simulink model "cdnlink_lb_wide_15a"  (Simulink 8.5)
settings: Solver=ode45  StartTime=0.0  StopTime=10.0  RelTol=1e-3
undefined symbols (not defined in the file): des, gcbh
(part 2 of 3)

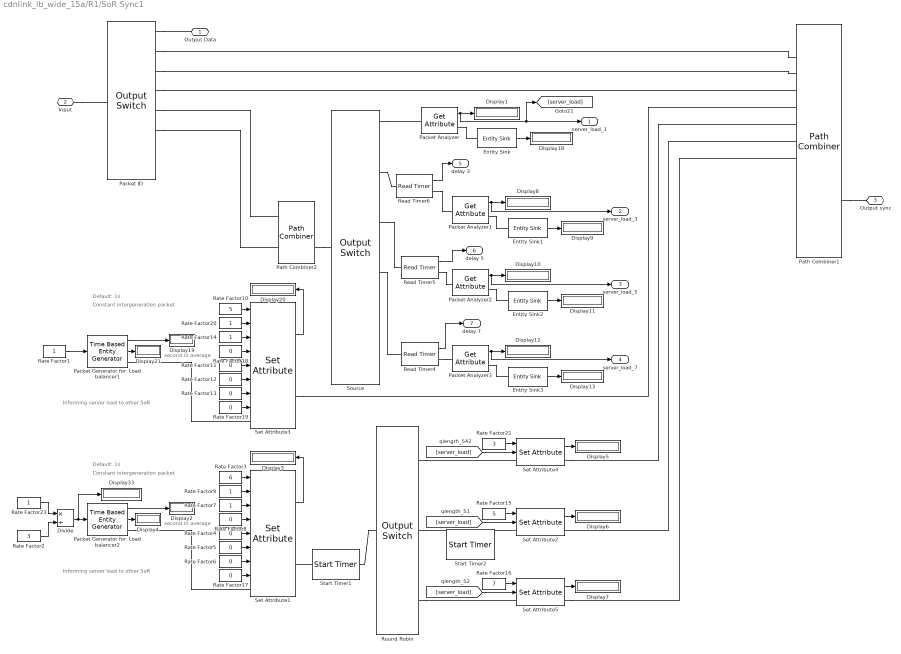
== system cdnlink_lb_wide_15a/R1/SoR Sync1 ==
  note: second in average
  note: Constant intergeneration packet
  note: Default: 1s
  note: Informing server load to other SoR
  note: second in average
  note: Constant intergeneration packet
  note: Default: 1s
  note: Informing server load to other SoR
  Display{1..13,18..21,33} (18 alike) : Display
  Divide : Product  Inputs=*/
  Entity Sink{,1..3} (4 alike) : EntitySink  StatNumberArrived=on
  Packet Analyzer : GetAttribute  AttributeName=av_load1  EvaluatedDefaultAttributeValue={ []}
      settings: OutputPortMap=o1
  Packet Analyzer1 : GetAttribute  AttributeName=server_load  EvaluatedDefaultAttributeValue={ []}
      settings: OutputPortMap=o1
  Packet Analyzer2 : GetAttribute  AttributeName=server_load  EvaluatedDefaultAttributeValue={ []}
      settings: OutputPortMap=o1
  Packet Analyzer3 : GetAttribute  AttributeName=server_load  EvaluatedDefaultAttributeValue={ []}
      settings: OutputPortMap=o1
  Packet Generator for  Load balancer1 : TimeBasedEntityGenerator  GenerateEntitiesUpon=Intergeneration time from port t  InitialSeed=6765331  Mean=0.05  EntityType=Standard  StatNumberDeparted=on  StatAverageIntergenerationTime=on
      settings: OutputPortMap=o0,o2
  Packet Generator for  Load balancer2 : TimeBasedEntityGenerator  GenerateEntitiesUpon=Intergeneration time from port t  InitialSeed=6765331  Mean=0.05  EntityType=Standard  StatNumberDeparted=on  StatAverageIntergenerationTime=on
      settings: OutputPortMap=o0,o2
  Packet ID : OutputSwitch  NumberOutputPorts=8  SwitchingCriterion=From attribute  AttributeName=packet_id
  Path Combiner1 : PathCombiner  NumberInputPorts=13  StatNumberDeparted=on
  Path Combiner2 : PathCombiner  NumberInputPorts=2  StatNumberDeparted=on
  Rate Factor{1,7,9,14,20,23} (6 alike) : Constant
  Rate Factor10 : Constant  Value=5
  Rate Factor{4..6,8,11..13,17..19} (10 alike) : Constant  Value=0
  Rate Factor15 : Constant  Value=5
  Rate Factor16 : Constant  Value=7
  Rate Factor2 : Constant  Value=3
  Rate Factor21 : Constant  Value=3
  Rate Factor3 : Constant  Value=6
  Read Timer4 : ReadTimer  TimerTag=id6  StatTimeElapsed=on
      settings: OutputPortMap=o2
  Read Timer5 : ReadTimer  TimerTag=id6  StatTimeElapsed=on
      settings: OutputPortMap=o2
  Read Timer6 : ReadTimer  TimerTag=id6  StatTimeElapsed=on
      settings: OutputPortMap=o2
  Round Robin : OutputSwitch  SwitchingCriterion=Round robin  AttributeName=source
  Set Attribute1 : SetAttribute  AttributeName=packet_id|reply|source|server_load|content_time|dest|hop_count|router_id  AttributeFrom=Signal port|Signal port|Signal port|Signal port|Signal port|Signal port|Signal port|Signal port  AttributeValue=1|1|1|1|1|1|1|1  AttributeTreatAsVector=1|1|1|1|1|1|1|1  StatNumberDeparted=on  EvaluatedAttributeValue={ [];[];[];[];[];[];[];[]}
      settings: InputPortMap=u0,u1,u2,u3,u4,u5,u6,u7
  Set Attribute2 : SetAttribute  AttributeName=dest|server_load  AttributeFrom=Signal port|Signal port  AttributeValue=1|1  AttributeTreatAsVector=1|1  StatNumberDeparted=on  EvaluatedAttributeValue={ [];[]}
      settings: InputPortMap=u0,u1
  Set Attribute3 : SetAttribute  AttributeName=packet_id|reply|source|server_load|content_time|dest|hop_count|router_id  AttributeFrom=Signal port|Signal port|Signal port|Signal port|Signal port|Signal port|Signal port|Signal port  AttributeValue=1|1|1|1|1|1|1|1  AttributeTreatAsVector=1|1|1|1|1|1|1|1  StatNumberDeparted=on  EvaluatedAttributeValue={ [];[];[];[];[];[];[];[]}
      settings: InputPortMap=u0,u1,u2,u3,u4,u5,u6,u7
  Set Attribute4 : SetAttribute  AttributeName=dest|server_load  AttributeFrom=Signal port|Signal port  AttributeValue=1|1  AttributeTreatAsVector=1|1  StatNumberDeparted=on  EvaluatedAttributeValue={ [];[]}
      settings: InputPortMap=u0,u1
  Set Attribute5 : SetAttribute  AttributeName=dest|server_load  AttributeFrom=Signal port|Signal port  AttributeValue=1|1  AttributeTreatAsVector=1|1  StatNumberDeparted=on  EvaluatedAttributeValue={ [];[]}
      settings: InputPortMap=u0,u1
  Source : OutputSwitch  NumberOutputPorts=11  SwitchingCriterion=From attribute  AttributeName=source
  Start Timer1 : StartTimer  TimerTag=id6
  Start Timer2 : StartTimer  TimerTag=id6
  Output Data : PMIOPort  Port=1  Side=Right
  Input : PMIOPort  Port=2  Side=Left
  Output sync : PMIOPort  Port=3  Side=Right
  server_load_1 : Outport
  server_load_3 : Outport  Port=2
  server_load_5 : Outport  Port=3
  server_load_7 : Outport  Port=4
  delay 3 : Outport  Port=5
  delay 5 : Outport  Port=6
  delay 7 : Outport  Port=7
  wires:
  Packet Generator for  Load balancer1/1 -> Display19/1
  Rate Factor14/1 -> Set Attribute3/3
  Rate Factor10/1 -> Set Attribute3/1
  Rate Factor20/1 -> Set Attribute3/2
  Packet Generator for  Load balancer1/2 -> Display21/1
  Rate Factor18/1 -> Set Attribute3/4
  Set Attribute3/1 -> Display20/1
  Rate Factor11/1 -> Set Attribute3/5
  Rate Factor12/1 -> Set Attribute3/6
  Rate Factor13/1 -> Set Attribute3/7
  Rate Factor1/1 -> Packet Generator for  Load balancer1/1
  Packet Analyzer/1 -> [server_load], server_load_1/1, Display1/1
  Entity Sink/1 -> Display18/1
  Packet Generator for  Load balancer2/1 -> Display2/1
  Rate Factor7/1 -> Set Attribute1/3
  Rate Factor3/1 -> Set Attribute1/1
  Rate Factor9/1 -> Set Attribute1/2
  Packet Generator for  Load balancer2/2 -> Display4/1
  Rate Factor8/1 -> Set Attribute1/4
  Set Attribute1/1 -> Display3/1
  Rate Factor4/1 -> Set Attribute1/5
  Rate Factor5/1 -> Set Attribute1/6
  Rate Factor6/1 -> Set Attribute1/7
  Rate Factor21/1 -> Set Attribute4/1
  Set Attribute4/1 -> Display5/1
  [server_load] -> Set Attribute4/2
  Rate Factor15/1 -> Set Attribute2/1
  Set Attribute2/1 -> Display6/1
  [server_load] -> Set Attribute2/2
  Rate Factor16/1 -> Set Attribute5/1
  Set Attribute5/1 -> Display7/1
  [server_load] -> Set Attribute5/2
  Packet Analyzer1/1 -> server_load_3/1, Display8/1
  Entity Sink1/1 -> Display9/1
  Packet Analyzer2/1 -> server_load_5/1, Display10/1
  Entity Sink2/1 -> Display11/1
  Packet Analyzer3/1 -> server_load_7/1, Display12/1
  Entity Sink3/1 -> Display13/1
  Rate Factor23/1 -> Divide/1
  Rate Factor2/1 -> Divide/2
  Divide/1 -> Packet Generator for  Load balancer2/1, Display33/1
  Rate Factor17/1 -> Set Attribute1/8
  Rate Factor19/1 -> Set Attribute3/8
  Read Timer6/1 -> delay 3/1
  Read Timer5/1 -> delay 5/1
  Read Timer4/1 -> delay 7/1
  connections:
  Packet Generator for  Load balancer1/RConn1 -- Set Attribute3/LConn1
  Packet ID/RConn5 -- Path Combiner2/LConn1
  Packet ID/RConn2 -- Path Combiner1/LConn2
  Packet ID/RConn3 -- Path Combiner1/LConn3
  Packet ID/RConn4 -- Path Combiner1/LConn4
  Set Attribute3/RConn1 -- Path Combiner1/LConn5
  Packet ID/RConn1 -- Output Data/RConn1
  Path Combiner1/RConn1 -- Output sync/RConn1
  Packet Analyzer/RConn1 -- Entity Sink/LConn1
  Source/RConn1 -- Packet Analyzer/LConn1
  Start Timer1/LConn1 -- Set Attribute1/RConn1
  Packet Generator for  Load balancer2/RConn1 -- Set Attribute1/LConn1
  Round Robin/RConn1 -- Set Attribute4/LConn1
  Round Robin/RConn2 -- Set Attribute2/LConn1
  Round Robin/RConn3 -- Set Attribute5/LConn1
  Packet Analyzer1/RConn1 -- Entity Sink1/LConn1
  Packet Analyzer2/RConn1 -- Entity Sink2/LConn1
  Packet Analyzer3/RConn1 -- Entity Sink3/LConn1
  Source/RConn5 -- Read Timer5/LConn1
  Path Combiner2/RConn1 -- Source/LConn1
  Packet ID/RConn6 -- Path Combiner2/LConn2
  Set Attribute4/RConn1 -- Path Combiner1/LConn6
  Path Combiner1/LConn7 -- Set Attribute2/RConn1
  Set Attribute5/RConn1 -- Path Combiner1/LConn8
  Input/RConn1 -- Packet ID/LConn1
  Round Robin/LConn1 -- Start Timer1/RConn1
  Read Timer4/RConn1 -- Packet Analyzer3/LConn1
  Source/RConn7 -- Read Timer4/LConn1
  Read Timer5/RConn1 -- Packet Analyzer2/LConn1
  Source/RConn3 -- Read Timer6/LConn1
  Read Timer6/RConn1 -- Packet Analyzer1/LConn1

== system cdnlink_lb_wide_15a/R3/ 1 ==
  note: Exponential Distribution
      | Service Rate Generator
  note: CDNlink-NS
  note: 830 packet/ second = 10 Mbps
      | for Router --> 500 Mbps = 830*10*5 = 41500
      | for Server --> 100 Mbps = 830*10 = 8300
  "  " : Subsystem  mask(Exponential Random Number Generator){seed=85274}
      mask prompts: seed "Initial seed"
      mask help: Output exponentially distributed random numbers with the input rate. Output is repeatable for a given seed.
      mask Display: disp('Exponential\n Distribution');
  Display1 : Display
  Display4 : Display
  Service time : Outport
  wires:
  "  "/1(Out1) -> Display1/1, Service time/1
  [router3] -> Display4/1, "  "/1(Arrival Rate)

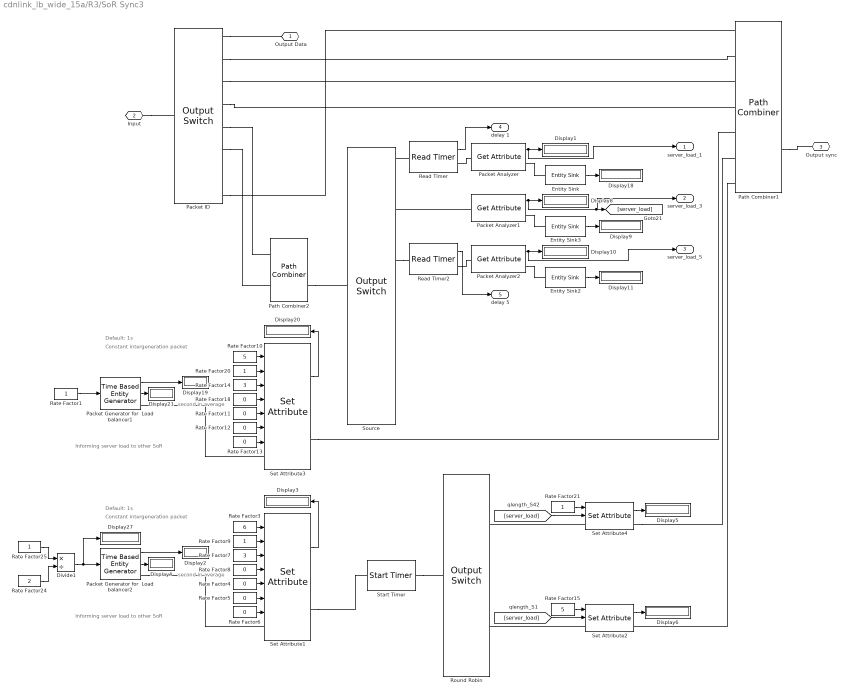
== system cdnlink_lb_wide_15a/R3/SoR Sync3 ==
  note: second in average
  note: Constant intergeneration packet
  note: Default: 1s
  note: Informing server load to other SoR
  note: second in average
  note: Constant intergeneration packet
  note: Default: 1s
  note: Informing server load to other SoR
  Display{1..6,8..11,18..21,27} (15 alike) : Display
  Divide1 : Product  Inputs=*/
  Entity Sink : EntitySink  StatNumberArrived=on
  Entity Sink2 : EntitySink  StatNumberArrived=on
  Entity Sink3 : EntitySink  StatNumberArrived=on
  Packet Analyzer : GetAttribute  AttributeName=server_load  EvaluatedDefaultAttributeValue={ []}
      settings: OutputPortMap=o1
  Packet Analyzer1 : GetAttribute  AttributeName=server_load  EvaluatedDefaultAttributeValue={ []}
      settings: OutputPortMap=o1
  Packet Analyzer2 : GetAttribute  AttributeName=server_load  EvaluatedDefaultAttributeValue={ []}
      settings: OutputPortMap=o1
  Packet Generator for  Load balancer1 : TimeBasedEntityGenerator  GenerateEntitiesUpon=Intergeneration time from port t  InitialSeed=6765331  Mean=0.05  EntityType=Standard  StatNumberDeparted=on  StatAverageIntergenerationTime=on
      settings: OutputPortMap=o0,o2
  Packet Generator for  Load balancer2 : TimeBasedEntityGenerator  GenerateEntitiesUpon=Intergeneration time from port t  InitialSeed=6765331  Mean=0.05  EntityType=Standard  StatNumberDeparted=on  StatAverageIntergenerationTime=on
      settings: OutputPortMap=o0,o2
  Packet ID : OutputSwitch  NumberOutputPorts=8  SwitchingCriterion=From attribute  AttributeName=packet_id
  Path Combiner1 : PathCombiner  NumberInputPorts=7  StatNumberDeparted=on
  Path Combiner2 : PathCombiner  NumberInputPorts=2  StatNumberDeparted=on
  Rate Factor{1,9,20..21,25} (5 alike) : Constant
  Rate Factor10 : Constant  Value=5
  Rate Factor{4..6,8,11..13,18} (8 alike) : Constant  Value=0
  Rate Factor14 : Constant  Value=3
  Rate Factor15 : Constant  Value=5
  Rate Factor24 : Constant  Value=2
  Rate Factor3 : Constant  Value=6
  Rate Factor7 : Constant  Value=3
  Read Timer : ReadTimer  TimerTag=id6  StatTimeElapsed=on
      settings: OutputPortMap=o2
  Read Timer2 : ReadTimer  TimerTag=id6  StatTimeElapsed=on
      settings: OutputPortMap=o2
  Round Robin : OutputSwitch  NumberOutputPorts=2  SwitchingCriterion=Round robin  AttributeName=source
  Set Attribute1 : SetAttribute  AttributeName=packet_id|reply|source|server_load|content_time|dest|hop_count  AttributeFrom=Signal port|Signal port|Signal port|Signal port|Signal port|Signal port|Signal port  AttributeValue=1|1|1|1|1|1|1  AttributeTreatAsVector=1|1|1|1|1|1|1  StatNumberDeparted=on  EvaluatedAttributeValue={ [];[];[];[];[];[];[]}
      settings: InputPortMap=u0,u1,u2,u3,u4,u5,u6
  Set Attribute2 : SetAttribute  AttributeName=dest|server_load  AttributeFrom=Signal port|Signal port  AttributeValue=1|1  AttributeTreatAsVector=1|1  StatNumberDeparted=on  EvaluatedAttributeValue={ [];[]}
      settings: InputPortMap=u0,u1
  Set Attribute3 : SetAttribute  AttributeName=packet_id|reply|source|server_load|content_time|dest|hop_count  AttributeFrom=Signal port|Signal port|Signal port|Signal port|Signal port|Signal port|Signal port  AttributeValue=1|1|1|1|1|1|1  AttributeTreatAsVector=1|1|1|1|1|1|1  StatNumberDeparted=on  EvaluatedAttributeValue={ [];[];[];[];[];[];[]}
      settings: InputPortMap=u0,u1,u2,u3,u4,u5,u6
  Set Attribute4 : SetAttribute  AttributeName=dest|server_load  AttributeFrom=Signal port|Signal port  AttributeValue=1|1  AttributeTreatAsVector=1|1  StatNumberDeparted=on  EvaluatedAttributeValue={ [];[]}
      settings: InputPortMap=u0,u1
  Source : OutputSwitch  NumberOutputPorts=11  SwitchingCriterion=From attribute  AttributeName=source
  Start Timer : StartTimer  TimerTag=id6
  Output Data : PMIOPort  Port=1  Side=Right
  Input : PMIOPort  Port=2  Side=Left
  Output sync : PMIOPort  Port=3  Side=Right
  server_load_1 : Outport
  server_load_3 : Outport  Port=2
  server_load_5 : Outport  Port=3
  delay 1 : Outport  Port=4
  delay 5 : Outport  Port=5
  wires:
  Packet Generator for  Load balancer1/1 -> Display19/1
  Rate Factor14/1 -> Set Attribute3/3
  Rate Factor10/1 -> Set Attribute3/1
  Rate Factor20/1 -> Set Attribute3/2
  Packet Generator for  Load balancer1/2 -> Display21/1
  Rate Factor18/1 -> Set Attribute3/4
  Set Attribute3/1 -> Display20/1
  Rate Factor11/1 -> Set Attribute3/5
  Rate Factor12/1 -> Set Attribute3/6
  Rate Factor13/1 -> Set Attribute3/7
  Rate Factor1/1 -> Packet Generator for  Load balancer1/1
  Packet Analyzer/1 -> server_load_1/1, Display1/1
  Entity Sink/1 -> Display18/1
  Packet Generator for  Load balancer2/1 -> Display2/1
  Rate Factor7/1 -> Set Attribute1/3
  Rate Factor3/1 -> Set Attribute1/1
  Rate Factor9/1 -> Set Attribute1/2
  Packet Generator for  Load balancer2/2 -> Display4/1
  Rate Factor8/1 -> Set Attribute1/4
  Set Attribute1/1 -> Display3/1
  Rate Factor4/1 -> Set Attribute1/5
  Rate Factor5/1 -> Set Attribute1/6
  Rate Factor6/1 -> Set Attribute1/7
  Rate Factor21/1 -> Set Attribute4/1
  Set Attribute4/1 -> Display5/1
  [server_load] -> Set Attribute4/2
  Rate Factor15/1 -> Set Attribute2/1
  Set Attribute2/1 -> Display6/1
  [server_load] -> Set Attribute2/2
  Packet Analyzer2/1 -> server_load_5/1, Display10/1
  Entity Sink2/1 -> Display11/1
  Packet Analyzer1/1 -> [server_load], server_load_3/1, Display8/1
  Entity Sink3/1 -> Display9/1
  Rate Factor25/1 -> Divide1/1
  Rate Factor24/1 -> Divide1/2
  Divide1/1 -> Packet Generator for  Load balancer2/1, Display27/1
  Read Timer/1 -> delay 1/1
  Read Timer2/1 -> delay 5/1
  connections:
  Input/RConn1 -- Packet ID/LConn1
  Packet Generator for  Load balancer1/RConn1 -- Set Attribute3/LConn1
  Packet ID/RConn5 -- Path Combiner2/LConn1
  Packet ID/RConn2 -- Path Combiner1/LConn2
  Packet ID/RConn3 -- Path Combiner1/LConn3
  Packet ID/RConn4 -- Path Combiner1/LConn4
  Set Attribute3/RConn1 -- Path Combiner1/LConn5
  Packet ID/RConn1 -- Output Data/RConn1
  Path Combiner1/RConn1 -- Output sync/RConn1
  Packet Analyzer/RConn1 -- Entity Sink/LConn1
  Read Timer/LConn1 -- Source/RConn1
  Start Timer/RConn1 -- Round Robin/LConn1
  Packet Generator for  Load balancer2/RConn1 -- Set Attribute1/LConn1
  Set Attribute4/LConn1 -- Round Robin/RConn1
  Set Attribute2/LConn1 -- Round Robin/RConn2
  Packet Analyzer2/RConn1 -- Entity Sink2/LConn1
  Packet Analyzer1/LConn1 -- Source/RConn3
  Source/RConn5 -- Read Timer2/LConn1
  Path Combiner2/RConn1 -- Source/LConn1
  Packet ID/RConn6 -- Path Combiner2/LConn2
  Path Combiner1/LConn7 -- Set Attribute2/RConn1
  Set Attribute4/RConn1 -- Path Combiner1/LConn6
  Packet Analyzer1/RConn1 -- Entity Sink3/LConn1
  Packet ID/RConn8 -- Path Combiner1/LConn1
  Set Attribute1/RConn1 -- Start Timer/LConn1
  Read Timer/RConn1 -- Packet Analyzer/LConn1
  Read Timer2/RConn1 -- Packet Analyzer2/LConn1

== system cdnlink_lb_wide_15a/S1/Atomic Subsystem ==
  In1 : Inport
  In2 : Inport  Port=2
  Divide : Product  Inputs=*/
  Out1 : Outport
  wires:
  In1/1 -> Divide/1
  Divide/1 -> Out1/1
  In2/1 -> Divide/2

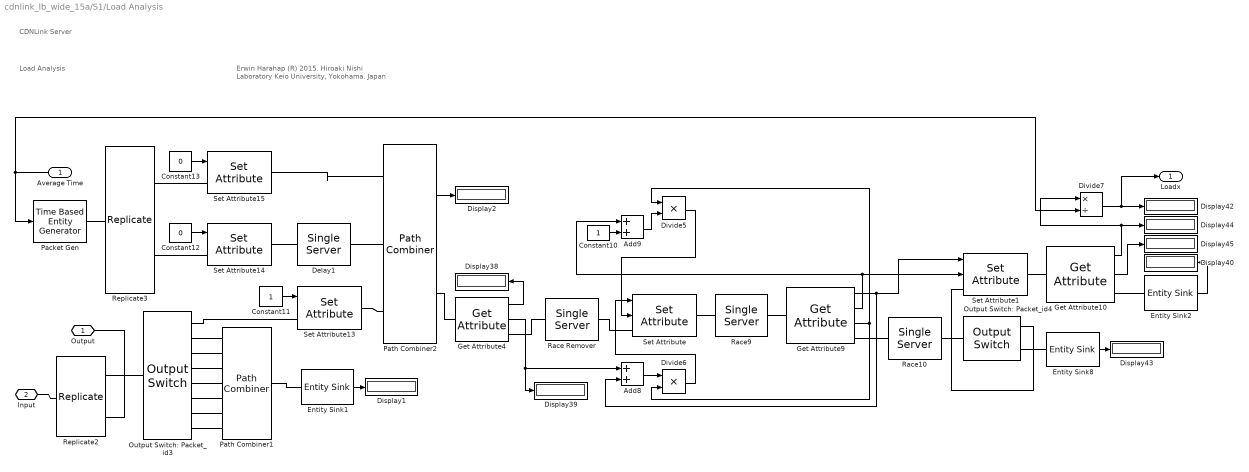
== system cdnlink_lb_wide_15a/S1/Load Analysis ==
  note: CDNLink Server
  note: Load Analysis
  note: Erwin Harahap
      | (R) 2015. Hiroaki Nishi Laboratory
      | Keio University, Yokohama.
      | Japan
  Average Time : Inport
  Add8 : Sum
  Add9 : Sum
  Constant10 : Constant
  Constant11 : Constant
  Constant12 : Constant  Value=0
  Constant13 : Constant  Value=0
  Delay1 : SingleServer  ServiceTime=0.05  AttributeName=ServiceTimeDNS
  Display{1..2,38..40,42..45} (9 alike) : Display
  Divide5 : Product  Inputs=**
  Divide6 : Product  Inputs=**
  Divide7 : Product  Inputs=*/
  Entity Sink1 : EntitySink  StatNumberArrived=on
  "Entity Sink2 " : EntitySink  StatNumberArrived=on
  Entity Sink8 : EntitySink  StatNumberArrived=on
  Get Attribute10 : GetAttribute  AttributeName=loadx|divider  AttributeMissing=Error|Error  AttributeDefaultValue=1|1  AttributeTreatAsVector=1|1  AttributeSendTiming=After entity departure|After entity departure  EvaluatedDefaultAttributeValue={ [];[]}
      settings: OutputPortMap=o1,o2
  Get Attribute4 : GetAttribute  AttributeName=content_time  StatNumberDeparted=on  EvaluatedDefaultAttributeValue={ []}
      settings: OutputPortMap=o0,o1
  Get Attribute9 : GetAttribute  AttributeName=content_time|divider|multiplier  AttributeMissing=Error|Error|Error  AttributeDefaultValue=1|1|1  AttributeTreatAsVector=1|1|1  AttributeSendTiming=After entity departure|After entity departure|After entity departure  EvaluatedDefaultAttributeValue={ [];[];[]}
      settings: OutputPortMap=o1,o2,o3
  Output Switch: Packet_id3 : OutputSwitch  NumberOutputPorts=8  SwitchingCriterion=From attribute  AttributeName=packet_id
  Output Switch: Packet_id4 : OutputSwitch  NumberOutputPorts=2  SwitchingCriterion=From attribute  AttributeName=switchx
  Packet Gen : TimeBasedEntityGenerator  GenerateEntitiesUpon=Intergeneration time from port t  Distribution=Uniform  Period=10  InitialSeed=1715331  Maximum=5  Mean=0.05  ResponseWhenBlocked=Error  EntityType=Standard
  Path Combiner1 : PathCombiner  NumberInputPorts=7
  Path Combiner2 : PathCombiner  StatNumberDeparted=on
  Race Remover : SingleServer  ServiceTime=0  AttributeName=ServiceTimeDNS
  Race10 : SingleServer  ServiceTime=0  AttributeName=ServiceTimeDNS
  Race9 : SingleServer  ServiceTime=0  AttributeName=ServiceTimeDNS
  Replicate2 : Replicate  NumberOutputPorts=2
  Replicate3 : Replicate  NumberOutputPorts=2
  "Set Attribute " : SetAttribute  AttributeName=content_time|divider  AttributeFrom=Signal port|Signal port  AttributeValue=0.5|1  AttributeTreatAsVector=1|1  EvaluatedAttributeValue={ [];[]}
      settings: InputPortMap=u0,u1
  Set Attribute1 : SetAttribute  AttributeName=loadx|divider  AttributeFrom=Signal port|Signal port  AttributeValue=0.5|1  AttributeTreatAsVector=1|1  EvaluatedAttributeValue={ [];[]}
      settings: InputPortMap=u0,u1
  Set Attribute13 : SetAttribute  AttributeName=multiplier|switchx  AttributeFrom=Signal port|Dialog  AttributeValue=0.5|2  AttributeTreatAsVector=1|1  EvaluatedAttributeValue={ [];2}
  Set Attribute14 : SetAttribute  AttributeName=multiplier|content_time|switchx  AttributeFrom=Signal port|Dialog|Dialog  AttributeValue=0.5|0|2  AttributeTreatAsVector=1|1|1  EvaluatedAttributeValue={ [];0;2}
  Set Attribute15 : SetAttribute  AttributeName=loadx1|content_time|multiplier|switchx  AttributeFrom=Signal port|Dialog|Dialog|Dialog  AttributeValue=0.5|0|1|1  AttributeTreatAsVector=1|1|1|1  EvaluatedAttributeValue={ [];0;1;1}
  Output : PMIOPort  Port=1  Side=Right
  Input : PMIOPort  Port=2  Side=Left
  Loadx : Outport
  wires:
  Divide6/1 -> "Set Attribute "/1
  Average Time/1 -> Divide7/2, Packet Gen/1
  Get Attribute4/1 -> Display38/1
  Get Attribute4/2 -> Add8/1, Display39/1
  "Entity Sink2 "/1 -> Display40/1
  Constant10/1 -> Add9/2
  Constant12/1 -> Set Attribute14/1
  Constant11/1 -> Set Attribute13/1
  Add9/1 -> Divide5/2
  Divide5/1 -> "Set Attribute "/2
  Add8/1 -> Divide6/1
  Constant13/1 -> Set Attribute15/1
  Get Attribute9/1 -> Set Attribute1/1, Add8/2
  Divide7/1 -> Display42/1, Loadx/1
  Get Attribute9/2 -> Add9/1, Set Attribute1/2
  Get Attribute9/3 -> Divide6/2, Divide5/1
  Entity Sink8/1 -> Display43/1
  Get Attribute10/1 -> Display44/1, Divide7/1
  Get Attribute10/2 -> Display45/1
  Entity Sink1/1 -> Display1/1
  Path Combiner2/1 -> Display2/1
  connections:
  Set Attribute1/RConn1 -- Get Attribute10/LConn1
  Get Attribute4/RConn1 -- Race Remover/LConn1
  Set Attribute13/RConn1 -- Path Combiner2/LConn3
  Replicate2/RConn1 -- Output Switch: Packet_id3/LConn1
  Race Remover/RConn1 -- "Set Attribute "/LConn1
  Output Switch: Packet_id4/RConn2 -- Entity Sink8/LConn1
  Output Switch: Packet_id3/RConn1 -- Set Attribute13/LConn1
  Race9/RConn1 -- Get Attribute9/LConn1
  Path Combiner2/LConn2 -- Delay1/RConn1
  Replicate3/RConn2 -- Set Attribute14/LConn1
  Race10/RConn1 -- Output Switch: Packet_id4/LConn1
  Replicate3/RConn1 -- Set Attribute15/LConn1
  Output Switch: Packet_id4/RConn1 -- Set Attribute1/LConn1
  Set Attribute14/RConn1 -- Delay1/LConn1
  Get Attribute9/RConn1 -- Race10/LConn1
  Get Attribute10/RConn1 -- "Entity Sink2 "/LConn1
  Set Attribute15/RConn1 -- Path Combiner2/LConn1
  Get Attribute4/LConn1 -- Path Combiner2/RConn1
  Input/RConn1 -- Replicate2/LConn1
  Output/RConn1 -- Replicate2/RConn2
  Packet Gen/RConn1 -- Replicate3/LConn1
  "Set Attribute "/RConn1 -- Race9/LConn1
  Path Combiner1/RConn1 -- Entity Sink1/LConn1
  Output Switch: Packet_id3/RConn2 -- Path Combiner1/LConn1
  Output Switch: Packet_id3/RConn3 -- Path Combiner1/LConn2
  Output Switch: Packet_id3/RConn4 -- Path Combiner1/LConn3
  Output Switch: Packet_id3/RConn5 -- Path Combiner1/LConn4
  Output Switch: Packet_id3/RConn6 -- Path Combiner1/LConn5
  Output Switch: Packet_id3/RConn7 -- Path Combiner1/LConn6
  Output Switch: Packet_id3/RConn8 -- Path Combiner1/LConn7

== system cdnlink_lb_wide_15a/S1/Load Control Module ==
  note: second in average
  note: Constant intergeneration packet
  note: Default: 1s
  note: Informing server load to other SoR
  Display19 : Display
  Display20 : Display
  Display21 : Display
  Packet Generator for  Load balancer1 : TimeBasedEntityGenerator  GenerateEntitiesUpon=Intergeneration time from port t  InitialSeed=6765331  Mean=0.05  EntityType=Standard  StatNumberDeparted=on  StatAverageIntergenerationTime=on
      settings: OutputPortMap=o0,o2
  Rate Factor1 : Constant
  Rate Factor10 : Constant  Value=7
  Rate Factor{11..13,18} (4 alike) : Constant  Value=0
  Rate Factor14 : Constant
  Rate Factor20 : Constant
  Set Attribute3 : SetAttribute  AttributeName=packet_id|reply|source|server_load|content_time|dest|hop_count  AttributeFrom=Signal port|Signal port|Signal port|Signal port|Signal port|Signal port|Signal port  AttributeValue=1|1|1|1|1|1|1  AttributeTreatAsVector=1|1|1|1|1|1|1  StatNumberDeparted=on  EvaluatedAttributeValue={ [];[];[];[];[];[];[]}
      settings: InputPortMap=u0,u1,u2,u3,u4,u5,u6
  Conn1 : PMIOPort  Port=1  Side=Right
  data 2 : Outport
  wires:
  Packet Generator for  Load balancer1/1 -> Display19/1
  Rate Factor14/1 -> Set Attribute3/3
  Rate Factor10/1 -> Set Attribute3/1
  Rate Factor20/1 -> Set Attribute3/2
  Packet Generator for  Load balancer1/2 -> Display21/1
  Rate Factor18/1 -> Set Attribute3/4
  Set Attribute3/1 -> data 2/1, Display20/1
  Rate Factor11/1 -> Set Attribute3/5
  Rate Factor12/1 -> Set Attribute3/6
  Rate Factor13/1 -> Set Attribute3/7
  Rate Factor1/1 -> Packet Generator for  Load balancer1/1
  connections:
  Packet Generator for  Load balancer1/RConn1 -- Set Attribute3/LConn1
  Set Attribute3/RConn1 -- Conn1/RConn1

== system cdnlink_lb_wide_15a/S3/Atomic Subsystem ==
  In1 : Inport
  In2 : Inport  Port=2
  Divide : Product  Inputs=*/
  Out1 : Outport
  wires:
  In1/1 -> Divide/1
  Divide/1 -> Out1/1
  In2/1 -> Divide/2

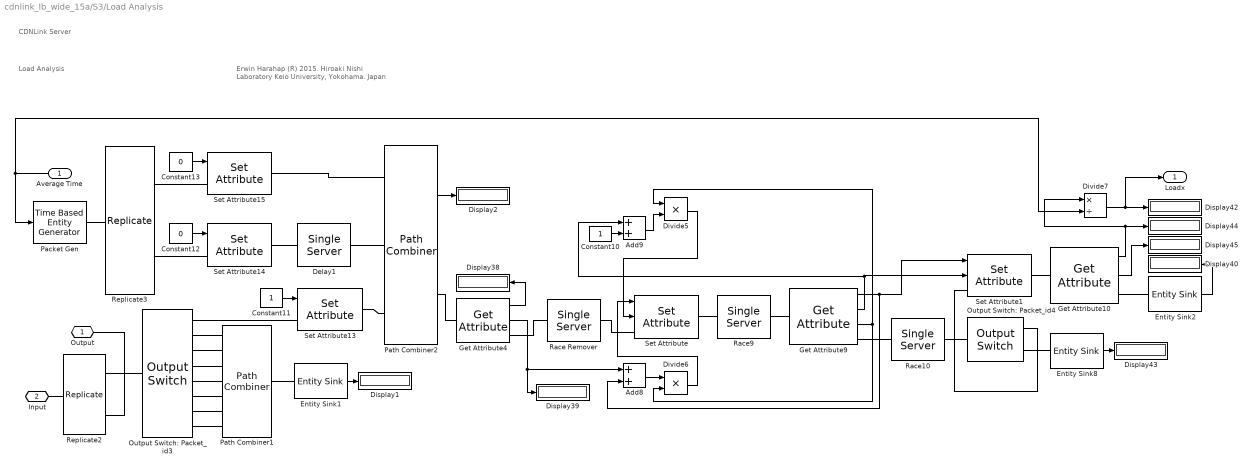
== system cdnlink_lb_wide_15a/S3/Load Analysis ==
  note: CDNLink Server
  note: Load Analysis
  note: Erwin Harahap
      | (R) 2015. Hiroaki Nishi Laboratory
      | Keio University, Yokohama.
      | Japan
  Average Time : Inport
  Add8 : Sum
  Add9 : Sum
  Constant10 : Constant
  Constant11 : Constant
  Constant12 : Constant  Value=0
  Constant13 : Constant  Value=0
  Delay1 : SingleServer  ServiceTime=0.05  AttributeName=ServiceTimeDNS
  Display{1..2,38..40,42..45} (9 alike) : Display
  Divide5 : Product  Inputs=**
  Divide6 : Product  Inputs=**
  Divide7 : Product  Inputs=*/
  Entity Sink1 : EntitySink  StatNumberArrived=on
  "Entity Sink2 " : EntitySink  StatNumberArrived=on
  Entity Sink8 : EntitySink  StatNumberArrived=on
  Get Attribute10 : GetAttribute  AttributeName=loadx|divider  AttributeMissing=Error|Error  AttributeDefaultValue=1|1  AttributeTreatAsVector=1|1  AttributeSendTiming=After entity departure|After entity departure  EvaluatedDefaultAttributeValue={ [];[]}
      settings: OutputPortMap=o1,o2
  Get Attribute4 : GetAttribute  AttributeName=content_time  StatNumberDeparted=on  EvaluatedDefaultAttributeValue={ []}
      settings: OutputPortMap=o0,o1
  Get Attribute9 : GetAttribute  AttributeName=content_time|divider|multiplier  AttributeMissing=Error|Error|Error  AttributeDefaultValue=1|1|1  AttributeTreatAsVector=1|1|1  AttributeSendTiming=After entity departure|After entity departure|After entity departure  EvaluatedDefaultAttributeValue={ [];[];[]}
      settings: OutputPortMap=o1,o2,o3
  Output Switch: Packet_id3 : OutputSwitch  NumberOutputPorts=8  SwitchingCriterion=From attribute  AttributeName=packet_id
  Output Switch: Packet_id4 : OutputSwitch  NumberOutputPorts=2  SwitchingCriterion=From attribute  AttributeName=switchx
  Packet Gen : TimeBasedEntityGenerator  GenerateEntitiesUpon=Intergeneration time from port t  Distribution=Uniform  Period=10  InitialSeed=1715331  Maximum=5  Mean=0.05  ResponseWhenBlocked=Error  EntityType=Standard
  Path Combiner1 : PathCombiner  NumberInputPorts=7
  Path Combiner2 : PathCombiner  StatNumberDeparted=on
  Race Remover : SingleServer  ServiceTime=0  AttributeName=ServiceTimeDNS
  Race10 : SingleServer  ServiceTime=0  AttributeName=ServiceTimeDNS
  Race9 : SingleServer  ServiceTime=0  AttributeName=ServiceTimeDNS
  Replicate2 : Replicate  NumberOutputPorts=2
  Replicate3 : Replicate  NumberOutputPorts=2
  "Set Attribute " : SetAttribute  AttributeName=content_time|divider  AttributeFrom=Signal port|Signal port  AttributeValue=0.5|1  AttributeTreatAsVector=1|1  EvaluatedAttributeValue={ [];[]}
      settings: InputPortMap=u0,u1
  Set Attribute1 : SetAttribute  AttributeName=loadx|divider  AttributeFrom=Signal port|Signal port  AttributeValue=0.5|1  AttributeTreatAsVector=1|1  EvaluatedAttributeValue={ [];[]}
      settings: InputPortMap=u0,u1
  Set Attribute13 : SetAttribute  AttributeName=multiplier|switchx  AttributeFrom=Signal port|Dialog  AttributeValue=0.5|2  AttributeTreatAsVector=1|1  EvaluatedAttributeValue={ [];2}
  Set Attribute14 : SetAttribute  AttributeName=multiplier|content_time|switchx  AttributeFrom=Signal port|Dialog|Dialog  AttributeValue=0.5|0|2  AttributeTreatAsVector=1|1|1  EvaluatedAttributeValue={ [];0;2}
  Set Attribute15 : SetAttribute  AttributeName=loadx1|content_time|multiplier|switchx  AttributeFrom=Signal port|Dialog|Dialog|Dialog  AttributeValue=0.5|0|1|1  AttributeTreatAsVector=1|1|1|1  EvaluatedAttributeValue={ [];0;1;1}
  Output : PMIOPort  Port=1  Side=Right
  Input : PMIOPort  Port=2  Side=Left
  Loadx : Outport
  wires:
  Divide6/1 -> "Set Attribute "/1
  Average Time/1 -> Divide7/2, Packet Gen/1
  Get Attribute4/1 -> Display38/1
  Get Attribute4/2 -> Add8/1, Display39/1
  "Entity Sink2 "/1 -> Display40/1
  Constant10/1 -> Add9/2
  Constant12/1 -> Set Attribute14/1
  Constant11/1 -> Set Attribute13/1
  Add9/1 -> Divide5/2
  Divide5/1 -> "Set Attribute "/2
  Add8/1 -> Divide6/1
  Constant13/1 -> Set Attribute15/1
  Get Attribute9/1 -> Set Attribute1/1, Add8/2
  Divide7/1 -> Display42/1, Loadx/1
  Get Attribute9/2 -> Add9/1, Set Attribute1/2
  Get Attribute9/3 -> Divide6/2, Divide5/1
  Entity Sink8/1 -> Display43/1
  Get Attribute10/1 -> Display44/1, Divide7/1
  Get Attribute10/2 -> Display45/1
  Entity Sink1/1 -> Display1/1
  Path Combiner2/1 -> Display2/1
  connections:
  Set Attribute1/RConn1 -- Get Attribute10/LConn1
  Get Attribute4/RConn1 -- Race Remover/LConn1
  Set Attribute13/RConn1 -- Path Combiner2/LConn3
  Replicate2/RConn1 -- Output Switch: Packet_id3/LConn1
  Race Remover/RConn1 -- "Set Attribute "/LConn1
  Output Switch: Packet_id4/RConn2 -- Entity Sink8/LConn1
  Output Switch: Packet_id3/RConn1 -- Set Attribute13/LConn1
  Race9/RConn1 -- Get Attribute9/LConn1
  Path Combiner2/LConn2 -- Delay1/RConn1
  Replicate3/RConn2 -- Set Attribute14/LConn1
  Race10/RConn1 -- Output Switch: Packet_id4/LConn1
  Replicate3/RConn1 -- Set Attribute15/LConn1
  Output Switch: Packet_id4/RConn1 -- Set Attribute1/LConn1
  Set Attribute14/RConn1 -- Delay1/LConn1
  Get Attribute9/RConn1 -- Race10/LConn1
  Get Attribute10/RConn1 -- "Entity Sink2 "/LConn1
  Set Attribute15/RConn1 -- Path Combiner2/LConn1
  Get Attribute4/LConn1 -- Path Combiner2/RConn1
  Input/RConn1 -- Replicate2/LConn1
  Output/RConn1 -- Replicate2/RConn2
  Packet Gen/RConn1 -- Replicate3/LConn1
  "Set Attribute "/RConn1 -- Race9/LConn1
  Path Combiner1/RConn1 -- Entity Sink1/LConn1
  Output Switch: Packet_id3/RConn2 -- Path Combiner1/LConn1
  Output Switch: Packet_id3/RConn3 -- Path Combiner1/LConn2
  Output Switch: Packet_id3/RConn4 -- Path Combiner1/LConn3
  Output Switch: Packet_id3/RConn5 -- Path Combiner1/LConn4
  Output Switch: Packet_id3/RConn6 -- Path Combiner1/LConn5
  Output Switch: Packet_id3/RConn7 -- Path Combiner1/LConn6
  Output Switch: Packet_id3/RConn8 -- Path Combiner1/LConn7

== system cdnlink_lb_wide_15a/S3/Load Control Module ==
  note: second in average
  note: Constant intergeneration packet
  note: Default: 1s
  note: Informing server load to other SoR
  Display19 : Display
  Display20 : Display
  Display21 : Display
  Packet Generator for  Load balancer1 : TimeBasedEntityGenerator  GenerateEntitiesUpon=Intergeneration time from port t  InitialSeed=6765331  Mean=0.05  EntityType=Standard  StatNumberDeparted=on  StatAverageIntergenerationTime=on
      settings: OutputPortMap=o0,o2
  Rate Factor1 : Constant
  Rate Factor10 : Constant  Value=7
  Rate Factor{11..13,18} (4 alike) : Constant  Value=0
  Rate Factor14 : Constant
  Rate Factor20 : Constant
  Set Attribute3 : SetAttribute  AttributeName=packet_id|reply|source|server_load|content_time|dest|hop_count  AttributeFrom=Signal port|Signal port|Signal port|Signal port|Signal port|Signal port|Signal port  AttributeValue=1|1|1|1|1|1|1  AttributeTreatAsVector=1|1|1|1|1|1|1  StatNumberDeparted=on  EvaluatedAttributeValue={ [];[];[];[];[];[];[]}
      settings: InputPortMap=u0,u1,u2,u3,u4,u5,u6
  Conn1 : PMIOPort  Port=1  Side=Right
  data 2 : Outport
  wires:
  Packet Generator for  Load balancer1/1 -> Display19/1
  Rate Factor14/1 -> Set Attribute3/3
  Rate Factor10/1 -> Set Attribute3/1
  Rate Factor20/1 -> Set Attribute3/2
  Packet Generator for  Load balancer1/2 -> Display21/1
  Rate Factor18/1 -> Set Attribute3/4
  Set Attribute3/1 -> data 2/1, Display20/1
  Rate Factor11/1 -> Set Attribute3/5
  Rate Factor12/1 -> Set Attribute3/6
  Rate Factor13/1 -> Set Attribute3/7
  Rate Factor1/1 -> Packet Generator for  Load balancer1/1
  connections:
  Packet Generator for  Load balancer1/RConn1 -- Set Attribute3/LConn1
  Set Attribute3/RConn1 -- Conn1/RConn1

== system cdnlink_lb_wide_15a/C1/Packet Request Generator/   ==
  note: Attention: The arrival rate
      | should not exceed the service
      | rate, which is 1 in this model.
  Arrival Rate : Inport
  Atpf5fce743_cd9b_464f_89a7_6e7eb441df80 : TimedToEventSignal
  Constant : Constant
  Divide : Product  Inputs=*/
  Math Function : Math  Operator=log  SaturateOnIntegerOverflow=on
  Product : Product  RndMeth=Zero
  Subtract : Sum  Inputs=+-
  Unary Minus : UnaryMinus
  Uniform Random Number : UniformRandomNumber  Minimum=0  Seed=seed  SampleTime=0
  Out1 : Outport
  wires:
  Math Function/1 -> Product/2
  Subtract/1 -> Math Function/1
  Uniform Random Number/1 -> Subtract/2
  Constant/1 -> Divide/1, Subtract/1
  Arrival Rate/1 -> Divide/2
  Divide/1 -> Product/1
  Product/1 -> Unary Minus/1
  Atpf5fce743_cd9b_464f_89a7_6e7eb441df80/1 -> Out1/1
  Unary Minus/1 -> Atpf5fce743_cd9b_464f_89a7_6e7eb441df80/1

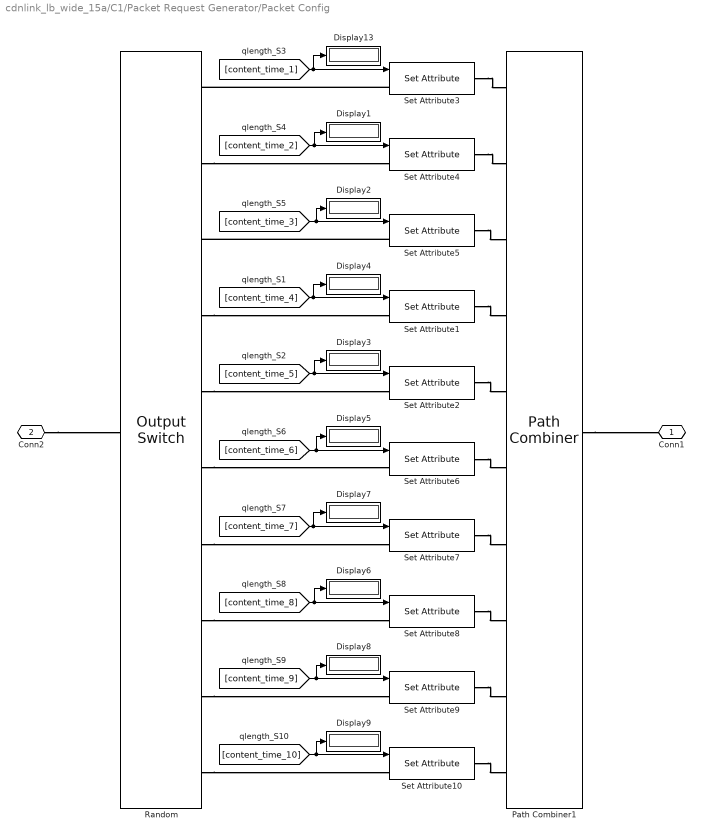
== system cdnlink_lb_wide_15a/C1/Packet Request Generator/Packet Config ==
  Display{1..9,13} (10 alike) : Display
  Path Combiner1 : PathCombiner  NumberInputPorts=10
  Random : OutputSwitch  NumberOutputPorts=10  SwitchingCriterion=Equiprobable  InitialSeed=13927  AttributeName=dest  InitialConditionsOpt=on
  Set Attribute1 : SetAttribute  AttributeName=content_id|content_time  AttributeFrom=Dialog|Signal port  AttributeValue=1|0.0475  AttributeTreatAsVector=1|1  EvaluatedAttributeValue={ 1;[]}
      settings: InputPortMap=u1
  Set Attribute{5..6,9..10} (4 alike) : SetAttribute  AttributeName=content_id|content_time  AttributeFrom=Dialog|Signal port  AttributeValue=3|0.3099  AttributeTreatAsVector=1|1  EvaluatedAttributeValue={ 3;[]}
      settings: InputPortMap=u1
  Set Attribute2 : SetAttribute  AttributeName=content_id|content_time  AttributeFrom=Dialog|Signal port  AttributeValue=2|0.5622  AttributeTreatAsVector=1|1  EvaluatedAttributeValue={ 2;[]}
      settings: InputPortMap=u1
  Set Attribute3 : SetAttribute  AttributeName=content_id|content_time  AttributeFrom=Dialog|Signal port  AttributeValue=1|0.0475  AttributeTreatAsVector=1|1  EvaluatedAttributeValue={ 1;[]}
      settings: InputPortMap=u1
  Set Attribute4 : SetAttribute  AttributeName=content_id|content_time  AttributeFrom=Dialog|Signal port  AttributeValue=2|0.5622  AttributeTreatAsVector=1|1  EvaluatedAttributeValue={ 2;[]}
      settings: InputPortMap=u1
  Set Attribute7 : SetAttribute  AttributeName=content_id|content_time  AttributeFrom=Dialog|Signal port  AttributeValue=1|0.0475  AttributeTreatAsVector=1|1  EvaluatedAttributeValue={ 1;[]}
      settings: InputPortMap=u1
  Set Attribute8 : SetAttribute  AttributeName=content_id|content_time  AttributeFrom=Dialog|Signal port  AttributeValue=2|0.5622  AttributeTreatAsVector=1|1  EvaluatedAttributeValue={ 2;[]}
      settings: InputPortMap=u1
  Conn1 : PMIOPort  Port=1  Side=Right
  Conn2 : PMIOPort  Port=2  Side=Left
  wires:
  [content_time_1] -> Display13/1, Set Attribute3/1
  [content_time_3] -> Display2/1, Set Attribute5/1
  [content_time_2] -> Display1/1, Set Attribute4/1
  [content_time_4] -> Display4/1, Set Attribute1/1
  [content_time_6] -> Display5/1, Set Attribute6/1
  [content_time_5] -> Display3/1, Set Attribute2/1
  [content_time_7] -> Display7/1, Set Attribute7/1
  [content_time_9] -> Display8/1, Set Attribute9/1
  [content_time_8] -> Display6/1, Set Attribute8/1
  [content_time_10] -> Display9/1, Set Attribute10/1
  connections:
  Conn2/RConn1 -- Random/LConn1
  Path Combiner1/RConn1 -- Conn1/RConn1
  Set Attribute3/RConn1 -- Path Combiner1/LConn1
  Set Attribute4/RConn1 -- Path Combiner1/LConn2
  Set Attribute5/RConn1 -- Path Combiner1/LConn3
  Set Attribute5/LConn1 -- Random/RConn3
  Set Attribute3/LConn1 -- Random/RConn1
  Random/RConn2 -- Set Attribute4/LConn1
  Random/RConn4 -- Set Attribute1/LConn1
  Random/RConn6 -- Set Attribute6/LConn1
  Random/RConn5 -- Set Attribute2/LConn1
  Random/RConn7 -- Set Attribute7/LConn1
  Random/RConn9 -- Set Attribute9/LConn1
  Random/RConn8 -- Set Attribute8/LConn1
  Random/RConn10 -- Set Attribute10/LConn1
  Set Attribute1/RConn1 -- Path Combiner1/LConn4
  Set Attribute2/RConn1 -- Path Combiner1/LConn5
  Set Attribute6/RConn1 -- Path Combiner1/LConn6
  Set Attribute7/RConn1 -- Path Combiner1/LConn7
  Set Attribute8/RConn1 -- Path Combiner1/LConn8
  Set Attribute9/RConn1 -- Path Combiner1/LConn9
  Set Attribute10/RConn1 -- Path Combiner1/LConn10

== system cdnlink_lb_wide_15a/C3/Packet Request Generator/   ==
  note: Attention: The arrival rate
      | should not exceed the service
      | rate, which is 1 in this model.
  Arrival Rate : Inport
  Atpf5fce743_cd9b_464f_89a7_6e7eb441df80 : TimedToEventSignal
  Constant : Constant
  Divide : Product  Inputs=*/
  Math Function : Math  Operator=log  SaturateOnIntegerOverflow=on
  Product : Product  RndMeth=Zero
  Subtract : Sum  Inputs=+-
  Unary Minus : UnaryMinus
  Uniform Random Number : UniformRandomNumber  Minimum=0  Seed=seed  SampleTime=0
  Out1 : Outport
  wires:
  Product/1 -> Unary Minus/1
  Math Function/1 -> Product/2
  Subtract/1 -> Math Function/1
  Uniform Random Number/1 -> Subtract/2
  Constant/1 -> Divide/1, Subtract/1
  Arrival Rate/1 -> Divide/2
  Divide/1 -> Product/1
  Unary Minus/1 -> Atpf5fce743_cd9b_464f_89a7_6e7eb441df80/1
  Atpf5fce743_cd9b_464f_89a7_6e7eb441df80/1 -> Out1/1

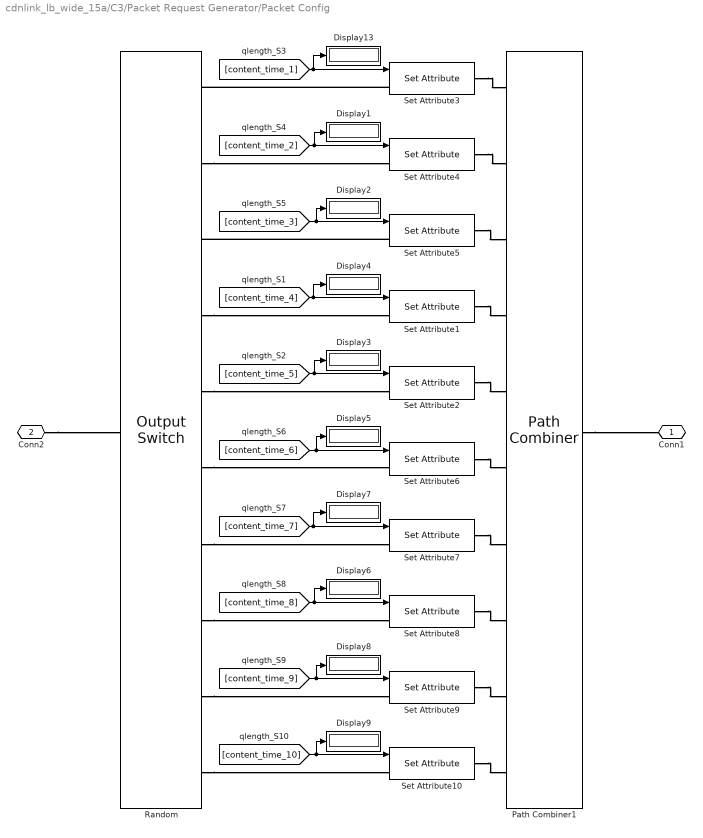
== system cdnlink_lb_wide_15a/C3/Packet Request Generator/Packet Config ==
  Display{1..9,13} (10 alike) : Display
  Path Combiner1 : PathCombiner  NumberInputPorts=10
  Random : OutputSwitch  NumberOutputPorts=10  SwitchingCriterion=Equiprobable  InitialSeed=13927  AttributeName=dest  InitialConditionsOpt=on
  Set Attribute1 : SetAttribute  AttributeName=content_id|content_time  AttributeFrom=Dialog|Signal port  AttributeValue=1|0.0475  AttributeTreatAsVector=1|1  EvaluatedAttributeValue={ 1;[]}
      settings: InputPortMap=u1
  Set Attribute{5..6,9..10} (4 alike) : SetAttribute  AttributeName=content_id|content_time  AttributeFrom=Dialog|Signal port  AttributeValue=3|0.3099  AttributeTreatAsVector=1|1  EvaluatedAttributeValue={ 3;[]}
      settings: InputPortMap=u1
  Set Attribute2 : SetAttribute  AttributeName=content_id|content_time  AttributeFrom=Dialog|Signal port  AttributeValue=2|0.5622  AttributeTreatAsVector=1|1  EvaluatedAttributeValue={ 2;[]}
      settings: InputPortMap=u1
  Set Attribute3 : SetAttribute  AttributeName=content_id|content_time  AttributeFrom=Dialog|Signal port  AttributeValue=1|0.0475  AttributeTreatAsVector=1|1  EvaluatedAttributeValue={ 1;[]}
      settings: InputPortMap=u1
  Set Attribute4 : SetAttribute  AttributeName=content_id|content_time  AttributeFrom=Dialog|Signal port  AttributeValue=2|0.5622  AttributeTreatAsVector=1|1  EvaluatedAttributeValue={ 2;[]}
      settings: InputPortMap=u1
  Set Attribute7 : SetAttribute  AttributeName=content_id|content_time  AttributeFrom=Dialog|Signal port  AttributeValue=1|0.0475  AttributeTreatAsVector=1|1  EvaluatedAttributeValue={ 1;[]}
      settings: InputPortMap=u1
  Set Attribute8 : SetAttribute  AttributeName=content_id|content_time  AttributeFrom=Dialog|Signal port  AttributeValue=2|0.5622  AttributeTreatAsVector=1|1  EvaluatedAttributeValue={ 2;[]}
      settings: InputPortMap=u1
  Conn1 : PMIOPort  Port=1  Side=Right
  Conn2 : PMIOPort  Port=2  Side=Left
  wires:
  [content_time_1] -> Display13/1, Set Attribute3/1
  [content_time_3] -> Display2/1, Set Attribute5/1
  [content_time_2] -> Display1/1, Set Attribute4/1
  [content_time_4] -> Display4/1, Set Attribute1/1
  [content_time_6] -> Display5/1, Set Attribute6/1
  [content_time_5] -> Display3/1, Set Attribute2/1
  [content_time_7] -> Display7/1, Set Attribute7/1
  [content_time_9] -> Display8/1, Set Attribute9/1
  [content_time_8] -> Display6/1, Set Attribute8/1
  [content_time_10] -> Display9/1, Set Attribute10/1
  connections:
  Conn2/RConn1 -- Random/LConn1
  Path Combiner1/RConn1 -- Conn1/RConn1
  Set Attribute3/RConn1 -- Path Combiner1/LConn1
  Set Attribute4/RConn1 -- Path Combiner1/LConn2
  Set Attribute5/RConn1 -- Path Combiner1/LConn3
  Set Attribute5/LConn1 -- Random/RConn3
  Set Attribute3/LConn1 -- Random/RConn1
  Random/RConn2 -- Set Attribute4/LConn1
  Random/RConn4 -- Set Attribute1/LConn1
  Random/RConn6 -- Set Attribute6/LConn1
  Random/RConn5 -- Set Attribute2/LConn1
  Random/RConn7 -- Set Attribute7/LConn1
  Random/RConn9 -- Set Attribute9/LConn1
  Random/RConn8 -- Set Attribute8/LConn1
  Random/RConn10 -- Set Attribute10/LConn1
  Set Attribute1/RConn1 -- Path Combiner1/LConn4
  Set Attribute2/RConn1 -- Path Combiner1/LConn5
  Set Attribute6/RConn1 -- Path Combiner1/LConn6
  Set Attribute7/RConn1 -- Path Combiner1/LConn7
  Set Attribute8/RConn1 -- Path Combiner1/LConn8
  Set Attribute9/RConn1 -- Path Combiner1/LConn9
  Set Attribute10/RConn1 -- Path Combiner1/LConn10

== system cdnlink_lb_wide_15a/R1/ 1/   ==
  note: Attention: The arrival rate
      | should not exceed the service
      | rate, which is 1 in this model.
  Arrival Rate : Inport
  Atpf5fce743_cd9b_464f_89a7_6e7eb441df80 : TimedToEventSignal
  Constant : Constant
  Divide : Product  Inputs=*/
  Math Function : Math  Operator=log  SaturateOnIntegerOverflow=on
  Product : Product  RndMeth=Zero
  Subtract : Sum  Inputs=+-
  Unary Minus : UnaryMinus
  Uniform Random Number : UniformRandomNumber  Minimum=0  Seed=seed  SampleTime=0
  Out1 : Outport
  wires:
  Product/1 -> Unary Minus/1
  Math Function/1 -> Product/2
  Subtract/1 -> Math Function/1
  Uniform Random Number/1 -> Subtract/2
  Constant/1 -> Divide/1, Subtract/1
  Arrival Rate/1 -> Divide/2
  Divide/1 -> Product/1
  Unary Minus/1 -> Atpf5fce743_cd9b_464f_89a7_6e7eb441df80/1
  Atpf5fce743_cd9b_464f_89a7_6e7eb441df80/1 -> Out1/1

== system cdnlink_lb_wide_15a/R3/ 1/   ==
  note: Attention: The arrival rate
      | should not exceed the service
      | rate, which is 1 in this model.
  Arrival Rate : Inport
  Atpf5fce743_cd9b_464f_89a7_6e7eb441df80 : TimedToEventSignal
  Constant : Constant
  Divide : Product  Inputs=*/
  Math Function : Math  Operator=log  SaturateOnIntegerOverflow=on
  Product : Product  RndMeth=Zero
  Subtract : Sum  Inputs=+-
  Unary Minus : UnaryMinus
  Uniform Random Number : UniformRandomNumber  Minimum=0  Seed=seed  SampleTime=0
  Out1 : Outport
  wires:
  Product/1 -> Unary Minus/1
  Math Function/1 -> Product/2
  Subtract/1 -> Math Function/1
  Uniform Random Number/1 -> Subtract/2
  Constant/1 -> Divide/1, Subtract/1
  Arrival Rate/1 -> Divide/2
  Divide/1 -> Product/1
  Unary Minus/1 -> Atpf5fce743_cd9b_464f_89a7_6e7eb441df80/1
  Atpf5fce743_cd9b_464f_89a7_6e7eb441df80/1 -> Out1/1
